simulink model "quad_copter_control"  (R2016b)
settings: Solver=VariableStepAuto  StartTime=0.0  StopTime=70  RelTol=1e-3  EnableMultiTasking=on
undefined symbols (not defined in the file): dcgain, get, InnerReferenceModel, Mixer, OptimalInnerController, OptimalOuterController, OuterReferenceModel, PitchRateModel, Ri, Ro, step_size, Ts
settings Model: Creator=tibo  LastModifiedBy=tibo
settings OptimizationCC: LifeSpan=inf
settings DebuggingCC: SFUnexpectedBacktrackingDiag=warning  SFNoUnconditionalDefaultTransitionDiag=warning  SFExecutionAtInitializationDiag=none
settings GRTTargetCC: TargetLangStandard=C89/C90 (ANSI)  GeneratePreprocessorConditionals=Disable all
settings ConfigComp: CovMetricSettings=dw  CovHtmlReporting=on  CovSaveCumulativeToWorkspaceVar=on  CovSaveSingleToWorkspaceVar=on  CovExternalEMLEnable=off

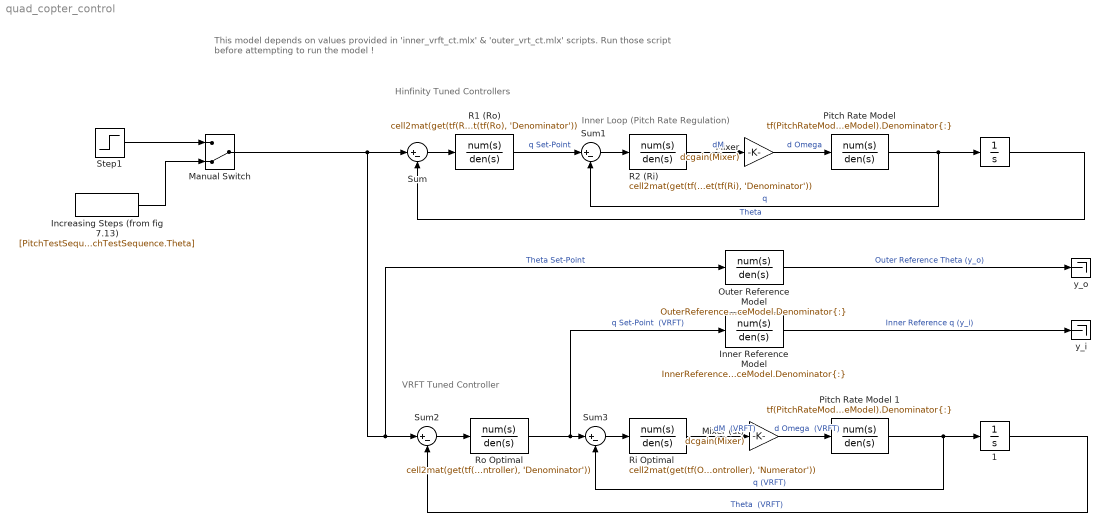
== system quad_copter_control ==
  note: Hinfinity Tuned Controllers
  note: VRFT Tuned Controller
  note: This model depends on values provided in 'inner_vrft_ct.mlx' & 'outer_vrt_ct.mlx' scripts.
      | Run those script before attempting to run the model !
  note: Inner Loop (Pitch Rate Regulation)
  " " : Integrator  ContinuousStateAttributes='PitchAngle'
  " 1" : Integrator  ContinuousStateAttributes='PitchAngle'
  Increasing Steps (from fig 7.13) : FromWorkspace  VariableName=[PitchTestSequence.Time, PitchTestSequence.Theta]  SampleTime=Ts  OutputAfterFinalValue=Holding final value
  Inner Reference Model : TransferFcn  Numerator=InnerReferenceModel.Numerator{:}  Denominator=InnerReferenceModel.Denominator{:}
  Manual Switch : ManualSwitch  CurrentSetting=0
  "Mixer " : Gain  Gain=dcgain(Mixer)
  Mixer (dt) : Gain  Gain=dcgain(Mixer)
  Outer Reference Model : TransferFcn  Numerator=OuterReferenceModel.Numerator{:}  Denominator=OuterReferenceModel.Denominator{:}
  "Pitch Rate Model " : TransferFcn  Numerator=tf(PitchRateModel).Numerator{:}  Denominator=tf(PitchRateModel).Denominator{:}  ContinuousStateAttributes='PitchRate'
  Pitch Rate Model 1 : TransferFcn  Numerator=tf(PitchRateModel).Numerator{:}  Denominator=tf(PitchRateModel).Denominator{:}  ContinuousStateAttributes='PitchRate'
  "R1 (Ro) " : TransferFcn  Numerator=cell2mat(get(tf(Ro), 'Numerator'))  Denominator=cell2mat(get(tf(Ro), 'Denominator'))
  "R2 (Ri) " : TransferFcn  Numerator=cell2mat(get(tf(Ri), 'Numerator'))  Denominator=cell2mat(get(tf(Ri), 'Denominator'))
  "Ri Optimal " : TransferFcn  Numerator=cell2mat(get(tf(OptimalInnerController), 'Numerator'))  Denominator=cell2mat(get(tf(OptimalInnerController), 'Numerator'))
  Ro Optimal : TransferFcn  Numerator=cell2mat(get(tf(OptimalOuterController), 'Numerator'))  Denominator=cell2mat(get(tf(OptimalOuterController), 'Denominator'))
  Step1 : Step  After=step_size  SampleTime=0
  Sum{,1..3} (4 alike) : Sum  Inputs=|+-
  y_i : Terminator
  y_o : Terminator
  wires:
  Sum/1 -> "R1 (Ro) "/1
  "R1 (Ro) "/1 -> Sum1/1  "q Set-Point"
  "R2 (Ri) "/1 -> "Mixer "/1  "dM"
  "Mixer "/1 -> "Pitch Rate Model "/1  "d Omega"
  "Pitch Rate Model "/1 -> Sum1/2, " "/1  "q"
  " "/1 -> Sum/2  "Theta"
  Increasing Steps (from fig 7.13)/1 -> Manual Switch/2
  Step1/1 -> Manual Switch/1
  Sum1/1 -> "R2 (Ri) "/1
  Sum2/1 -> Ro Optimal/1
  Ro Optimal/1 -> Inner Reference Model/1, Sum3/1  "q Set-Point  (VRFT)"
  "Ri Optimal "/1 -> Mixer (dt)/1  "dM  (VRFT)"
  Mixer (dt)/1 -> Pitch Rate Model 1/1  "d Omega  (VRFT)"
  Pitch Rate Model 1/1 -> " 1"/1, Sum3/2  "q (VRFT)"
  " 1"/1 -> Sum2/2  "Theta  (VRFT)"
  Sum3/1 -> "Ri Optimal "/1
  Outer Reference Model/1 -> y_o/1  "Outer Reference Theta (y_o)"
  Inner Reference Model/1 -> y_i/1  "Inner Reference q (y_i)"
  Manual Switch/1 -> Outer Reference Model/1, Sum2/1, Sum/1  "Theta Set-Point"
